simulink model "flightControlSystem"  (R2020b)
settings: Solver=ode3  StartTime=0  StopTime=TFinal  FixedStep=Ts  RelTol=1e-3  EnableMultiTasking=on
undefined symbols (not defined in the file): codertarget, Controller, DiscIntNeverNeededParam, Discrete, Estimator, g, gray, init, Rec, SDTV, Sensors, Time, Ts, var_acc_angle_N, var_bias_gyr_N, var_gyro_p_N, Vehicle
libraries: simulink x43, pid_lib x4, ctrlSharedLib x4, visiontransforms x4, sharedtransform x3, eeGeneralControl x2, visionstatistics x2, visionconversions x2, dspindex x2, dspbuff3 x1, uavalgslib x1, visiontextngfix x1
(part 3 of 3)

== system flightControlSystem/Flight Control System/State Estimator/XY Position Estimator/EstimatorXYPosition ==
  note: Switching from orientationControl to Position
      | control reset the current world position estimate
      | (happens when using no markers)
  dxy_estimin : Inport
  orient_estimin : Inport  Port=2  SampleTime=Ts
  controlModePosVSOrient_flagin : Inport  Port=3
  dz_estimin : Inport  Port=4
  Math Function : Math  Operator=transpose  SignedPower=on  SaturateOnIntegerOverflow=on
  Mux2 : Mux  Inputs=2
  Product : Product  Multiplication=Matrix(*)
  Rotation Angles to Direction Cosine Matrix : sharedtransform/Rotation Angles to Direction Cosine Matrix  rotationOrder=ZYX  aMode=aMode
      settings: SourceProductBaseCode=AE,PW,MT,UV,VE,VP
  SelectdXY : Selector  InputPortWidth=3  IndexOptions=Index vector (dialog)  Indices=[1 2]  OutputSizes=1
  SimplyIntegrateVelocity : DiscreteIntegrator  ExternalReset=rising  SampleTime=Ts  ICPrevOutput=DiscIntNeverNeededParam  ICPrevScaledInput=DiscIntNeverNeededParam
  XY_estimout : Outport  VectorParamsAs1DForOutWhenUnconnected=off
  wires:
  controlModePosVSOrient_flagin/1 -> SimplyIntegrateVelocity/2
  Product/1 -> SelectdXY/1
  Mux2/1 -> Product/2
  dz_estimin/1 -> Mux2/2
  SimplyIntegrateVelocity/1 -> XY_estimout/1
  dxy_estimin/1 -> Mux2/1
  orient_estimin/1 -> Rotation Angles to Direction Cosine Matrix/1
  Rotation Angles to Direction Cosine Matrix/1 -> Math Function/1
  SelectdXY/1 -> SimplyIntegrateVelocity/1
  Math Function/1 -> Product/1

== system flightControlSystem/Flight Control System/State Estimator/SensorPreprocessing/Temperature Compensation/Triggered Subsystem ==
  In1 : Inport
  Trigger : TriggerPort  TriggerType=either  VariantControl=Variant
  Out1 : Outport
  wires:
  In1/1 -> Out1/1

== system flightControlSystem/Flight Control System/State Estimator/XY Position Estimator/EstimatorVelocity/AccelerationHandling ==
  dxy_estimin : Inport
  sensorIMU_datin : Inport  Port=2
  orient_estimin : Inport  Port=3
  Z_estimin : Inport  Port=4
  Add : Sum  Inputs=-+
  Bus Selector1 : BusSelector  OutputSignals=ddx,ddy,ddz
  Deactivate Acceleration If OF is not used due to low altitude : simulink/Logic and Bit Operations/Compare To Constant  relop=<=  const=Estimator.pos.opticalFlowZMax  OutDataTypeStr=boolean
  Logical Operator : Logic  Operator=OR  AllPortsSameDT=off  OutDataTypeStr=boolean
  Mux6 : Mux  Inputs=3
  Product : Product  Inputs=3
  Product1 : Product  Multiplication=Matrix(*)
  Rotation Angles to Direction Cosine Matrix : sharedtransform/Rotation Angles to Direction Cosine Matrix  rotationOrder=ZYX  aMode=aMode
      settings: SourceProductBaseCode=AE,PW,MT,UV,VE,VP
  SelectPlanarddxy : Selector  InputPortWidth=3  IndexOptions=Index vector (dialog)  Indices=[1 2]  OutputSizes=1
  Selector : Selector  InputPortWidth=2  IndexOptions=Index vector (dialog)  Indices=1  OutputSizes=1
  Selector1 : Selector  InputPortWidth=2  IndexOptions=Index vector (dialog)  Indices=2  OutputSizes=1
  do not use acc if optical flow never available (Note OF@60Hz but ZOH to 200!) : simulink/Logic and Bit Operations/Compare To Constant  relop=~=  const=0  OutDataTypeStr=boolean
  do not use acc if optical flow never available (Note OF@60Hz but ZOH to 200!)1 : simulink/Logic and Bit Operations/Compare To Constant  relop=~=  const=0  OutDataTypeStr=boolean
  gainaccinput1 : Gain  OutDataTypeStr=single
  gravity : Constant  Value=[0 0 -g]
  acceleration_world : Outport  OutDataTypeStr=single  VectorParamsAs1DForOutWhenUnconnected=off
  wires:
  do not use acc if optical flow never available (Note OF@60Hz but ZOH to 200!)1/1 -> Logical Operator/2
  do not use acc if optical flow never available (Note OF@60Hz but ZOH to 200!)/1 -> Logical Operator/1
  Logical Operator/1 -> Product/1
  Selector1/1 -> do not use acc if optical flow never available (Note OF@60Hz but ZOH to 200!)1/1
  Selector/1 -> do not use acc if optical flow never available (Note OF@60Hz but ZOH to 200!)/1
  dxy_estimin/1 -> Selector1/1, Selector/1
  Product/1 -> acceleration_world/1
  Deactivate Acceleration If OF is not used due to low altitude/1 -> Product/3
  Z_estimin/1 -> Deactivate Acceleration If OF is not used due to low altitude/1
  Add/1 -> SelectPlanarddxy/1
  Product1/1 -> Add/1
  gravity/1 -> Product1/2
  SelectPlanarddxy/1 -> gainaccinput1/1
  Bus Selector1/3 -> Mux6/3  "<ddz>"
  Bus Selector1/1 -> Mux6/1  "<ddx>"
  sensorIMU_datin/1 -> Bus Selector1/1
  Mux6/1 -> Add/2
  Bus Selector1/2 -> Mux6/2  "<ddy>"
  orient_estimin/1 -> Rotation Angles to Direction Cosine Matrix/1
  Rotation Angles to Direction Cosine Matrix/1 -> Product1/1
  gainaccinput1/1 -> Product/2

== system flightControlSystem/Flight Control System/State Estimator/XY Position Estimator/EstimatorVelocity/Angular velocity compensation for optical flow ==
  note: Optical flow readings are affected by both linear and angular velocity of the drone. We need to subtract the effect of angular velocity before using the flow data
  z_estimate : Inport
  Angular velocity w/o bias : Inport  Port=2
  Abs : Abs
  Data Type Conversion : DataTypeConversion
  Demux : Demux  Outputs=2
  Gain1 : Gain  Gain=-1
  Mux : Mux  Inputs=2
  Selector : Selector  InputPortWidth=3  IndexOptions=Index vector (dialog)  Indices=[1 2]  OutputSizes=1
  prod : Product  Inputs=**
  angular velocity correction : Outport
  wires:
  Gain1/1 -> Mux/1
  Mux/1 -> Data Type Conversion/1
  Demux/2 -> Gain1/1
  Data Type Conversion/1 -> angular velocity correction/1
  prod/1 -> Demux/1
  z_estimate/1 -> Abs/1
  Demux/1 -> Mux/2
  Selector/1 -> prod/2
  Abs/1 -> prod/1
  Angular velocity w/o bias/1 -> Selector/1

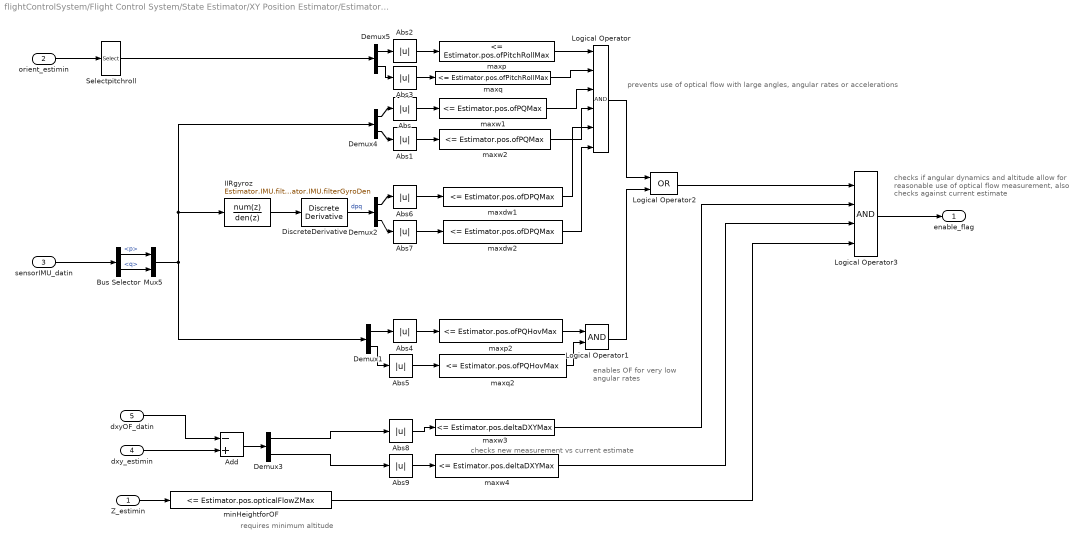
== system flightControlSystem/Flight Control System/State Estimator/XY Position Estimator/EstimatorVelocity/DataHandling ==
  note: prevents use of optical flow with large angles, angular rates or accelerations
  note: enables OF for very
      | low angular rates
  note: checks if angular dynamics and altitude allow for
      | reasonable use of optical flow measurement,
      | also checks against current estimate
  note: checks new measurement vs current estimate
  note: requires minimum altitude
  Z_estimin : Inport
  orient_estimin : Inport  Port=2
  sensorIMU_datin : Inport  Port=3
  dxy_estimin : Inport  Port=4
  dxyOF_datin : Inport  Port=5
  Abs{,1..9} (10 alike) : Abs
  Add : Sum  Inputs=-+
  Bus Selector : BusSelector  OutputSignals=p,q
  Demux{1..5} (5 alike) : Demux  Outputs=2
  DiscreteDerivative : simulink/Discrete/Discrete Derivative  gainval=1.0  ICPrevScaledInput=0.0  OutMin=[]  OutMax=[]  OutDataType=fixdt(1, 16)  OutScaling=2^-10  DoSatur=off
  IIRgyroz : DiscreteFilter  Numerator=Estimator.IMU.filterGyroNum  Denominator=Estimator.IMU.filterGyroDen
  Logical Operator : Logic  Inputs=6  AllPortsSameDT=off  OutDataTypeStr=boolean
  Logical Operator1 : Logic  AllPortsSameDT=off  OutDataTypeStr=boolean
  Logical Operator2 : Logic  Operator=OR  AllPortsSameDT=off  OutDataTypeStr=boolean
  Logical Operator3 : Logic  Inputs=4  AllPortsSameDT=off  OutDataTypeStr=boolean
  Mux5 : Mux  Inputs=2
  Selectpitchroll : Selector  InputPortWidth=3  IndexOptions=Index vector (dialog)  Indices=[2 3]  OutputSizes=1
  maxdw1 : simulink/Logic and Bit Operations/Compare To Constant  relop=<=  const=Estimator.pos.ofDPQMax  OutDataTypeStr=boolean
  maxdw2 : simulink/Logic and Bit Operations/Compare To Constant  relop=<=  const=Estimator.pos.ofDPQMax  OutDataTypeStr=boolean
  maxp : simulink/Logic and Bit Operations/Compare To Constant  relop=<=  const=Estimator.pos.ofPitchRollMax  OutDataTypeStr=boolean
  maxp2 : simulink/Logic and Bit Operations/Compare To Constant  relop=<=  const=Estimator.pos.ofPQHovMax  OutDataTypeStr=boolean
  maxq : simulink/Logic and Bit Operations/Compare To Constant  relop=<=  const=Estimator.pos.ofPitchRollMax  OutDataTypeStr=boolean
  maxq2 : simulink/Logic and Bit Operations/Compare To Constant  relop=<=  const=Estimator.pos.ofPQHovMax  OutDataTypeStr=boolean
  maxw1 : simulink/Logic and Bit Operations/Compare To Constant  relop=<=  const=Estimator.pos.ofPQMax  OutDataTypeStr=boolean
  maxw2 : simulink/Logic and Bit Operations/Compare To Constant  relop=<=  const=Estimator.pos.ofPQMax  OutDataTypeStr=boolean
  maxw3 : simulink/Logic and Bit Operations/Compare To Constant  relop=<=  const=Estimator.pos.deltaDXYMax  OutDataTypeStr=boolean
  maxw4 : simulink/Logic and Bit Operations/Compare To Constant  relop=<=  const=Estimator.pos.deltaDXYMax  OutDataTypeStr=boolean
  minHeightforOF : simulink/Logic and Bit Operations/Compare To Constant  relop=<=  const=Estimator.pos.opticalFlowZMax  OutDataTypeStr=boolean
  enable_flag : Outport  VectorParamsAs1DForOutWhenUnconnected=off
  wires:
  minHeightforOF/1 -> Logical Operator3/4
  IIRgyroz/1 -> DiscreteDerivative/1
  Mux5/1 -> Demux1/1, Demux4/1, IIRgyroz/1
  maxw4/1 -> Logical Operator3/3
  maxw3/1 -> Logical Operator3/2
  dxyOF_datin/1 -> Add/1
  Demux3/2 -> Abs9/1
  Demux3/1 -> Abs8/1
  dxy_estimin/1 -> Add/2
  Add/1 -> Demux3/1
  Abs9/1 -> maxw4/1
  Abs8/1 -> maxw3/1
  Logical Operator2/1 -> Logical Operator3/1
  Logical Operator3/1 -> enable_flag/1
  DiscreteDerivative/1 -> Demux2/1  "dpq"
  Demux2/2 -> Abs7/1
  Demux2/1 -> Abs6/1
  Abs7/1 -> maxdw2/1
  Abs6/1 -> maxdw1/1
  Logical Operator1/1 -> Logical Operator2/2
  Demux1/2 -> Abs5/1
  Demux1/1 -> Abs4/1
  Abs5/1 -> maxq2/1
  Abs4/1 -> maxp2/1
  Abs3/1 -> maxq/1
  Abs2/1 -> maxp/1
  Demux4/2 -> Abs1/1
  Demux4/1 -> Abs/1
  Abs1/1 -> maxw2/1
  Abs/1 -> maxw1/1
  Z_estimin/1 -> minHeightforOF/1
  Logical Operator/1 -> Logical Operator2/1
  maxw1/1 -> Logical Operator/3
  Bus Selector/1 -> Mux5/1  "<p>"
  Selectpitchroll/1 -> Demux5/1
  sensorIMU_datin/1 -> Bus Selector/1
  maxq2/1 -> Logical Operator1/2
  Bus Selector/2 -> Mux5/2  "<q>"
  maxp/1 -> Logical Operator/1
  maxw2/1 -> Logical Operator/4
  orient_estimin/1 -> Selectpitchroll/1
  maxdw1/1 -> Logical Operator/5
  maxdw2/1 -> Logical Operator/6
  maxq/1 -> Logical Operator/2
  Demux5/1 -> Abs2/1
  Demux5/2 -> Abs3/1
  maxp2/1 -> Logical Operator1/1

== system flightControlSystem/Flight Control System/State Estimator/XY Position Estimator/EstimatorVelocity/XY velocity w//o angular velocity compensation ==
  note: Optical flow raw readings are converted to velocity in m/s based on the estimated altitude
  optical_flow : Inport
  z_estimate : Inport  Port=2
  " " : Product  Inputs=**
  Compare To Constant : simulink/Logic and Bit Operations/Compare To Constant  relop=<  const=200*4  OutDataTypeStr=boolean
  Counter Free-Running : simulink/Sources/Counter Free-Running  NumBits=32  tsamp=-1
  Gain : Gain  Gain=-1
  Select dxy : Selector  InputPortWidth=3  IndexOptions=Index vector (dialog)  Indices=[1 2]  OutputSizes=1
  Switch : Switch  Criteria=u2 > Threshold
  opticalFlowErrorCorrect : Gain  Gain=1.15
  optical_flow_dx_dy : Outport
  wires:
  Select dxy/1 -> optical_flow_dx_dy/1  "optical_flow_dx_dy"
  " "/1 -> opticalFlowErrorCorrect/1
  opticalFlowErrorCorrect/1 -> Switch/3
  Gain/1 -> " "/2
  Switch/1 -> Select dxy/1
  Counter Free-Running/1 -> Compare To Constant/1
  Compare To Constant/1 -> Switch/2
  optical_flow/1 -> " "/1, Switch/1
  z_estimate/1 -> Gain/1

== matlab function flightControlSystem/Image Processing System/MATLAB Function ==
  data: lines_struc input; x output; y output
function [x,y]  = create_line_matrix(lines_struc)
    % convert lines struct to matrix
    coder.varsize('lines');
    lines = zeros(20,6);
    if size(lines_struc,1)<=20
        for i=1:size(lines_struc,1)
            lines(i,1) = lines_struc(i,1);
            lines(i,2) = lines_struc(i,2);
            lines(i,3) = lines_struc(i,3);
            lines(i,4) = lines_struc(i,4);
            line_vector = [lines(i,3)-lines(i,1), lines(i,4)-lines(i,2)];
            angle_slop = calculate_slop_angle(line_vector);
            lines(i,5) = angle_slop;
            lines(i,6) = sqrt((lines(i,3)-lines(i,1))^2+(lines(i,4)-lines(i,2))^2);
        end
    else
        for i=1:20
            lines(i,1) = lines_struc(i,1);
            lines(i,2) = lines_struc(i,2);
            lines(i,3) = lines_struc(i,3);
            lines(i,4) = lines_struc(i,4);
            line_vector = [lines(i,3)-lines(i,1), lines(i,4)-lines(i,2)];
            angle_slop = calculate_slop_angle(line_vector);
            lines(i,5) = angle_slop;
            lines(i,6) = sqrt((lines(i,3)-lines(i,1))^2+(lines(i,4)-lines(i,2))^2);
        end
    end
    
    %delete short line
    short_line_index = find(lines(:,6)<15);
    all_index = [1:1:20];
    all_index = all_index';
    long_line_index = setdiff(all_index,short_line_index,'rows');
    nline = size(long_line_index,1);
    new_lines = zeros(nline,6);
    new_lines = lines(long_line_index,:);
    lines = new_lines;
    %
    
    % detect lines to merge
    coder.varsize('parallel_line');
    parallel_line = zeros(20,8);
    parallel_line_insert_idx = 1;
    slop_value = unique(lines(:,5)); %OK
    coder.varsize('slop_value_to_checkmerge');
    slop_value_to_checkmerge = zeros(20,1); 
    slop_value_to_checkmerge_insert_idx = 1;
    coder.varsize('checked_slop');
    checked_slop = zeros(20,1);
    checked_slop_insert_idx = 1;
    if size(slop_value,1)>0
        for j = 1:size(slop_value,1)
            slop = slop_value(j);
            index_lines = find(abs(lines(:,5)-slop)<10);
            if size(index_lines,1)==2 && ~any(ismember(lines(index_lines,5),checked_slop))
                parallel_line(parallel_line_insert_idx,1:8) = [lines(index_lines(1),1:4),lines(index_lines(2),1:4)];
                parallel_line_insert_idx = parallel_line_insert_idx + 1 ;
            elseif size(index_lines,1)>2 && ~any(ismember(lines(index_lines,5),checked_slop))
                slop_value_to_checkmerge(slop_value_to_checkmerge_insert_idx) = slop;
                slop_value_to_checkmerge_insert_idx = slop_value_to_checkmerge_insert_idx+1;
            end
            checked_slop(checked_slop_insert_idx) = slop;
            checked_slop_insert_idx = checked_slop_insert_idx+1;
        end
    end
    slop_value_to_checkmerge = find(slop_value_to_checkmerge(:)~=0);
    %

    possible_interdistance = 100;
    if size(slop_value_to_checkmerge,1)>0
        for j=1:size(slop_value_to_checkmerge,1)
            slop = slop_value_to_checkmerge(j);
            index_lines = find(abs(lines(:,5)-slop)<10);
            %index_lines (maybe not only 2)
            middle_point_coordinates = [(lines(index_lines,1)+lines(index_lines,3))/2, (lines(index_lines,2)+lines(index_lines,4))/2];
            coder.varsize('merge_line_idx');
            merge_line_idx = zeros(20,2);
            merge_line_insert_idx = 1;
            for k=1:size(middle_point_coordinates,1)-1
                for h=k+1:size(middle_point_coordinates,1)
                    p1 = middle_point_coordinates(k,:);
                    p2 = middle_point_coordinates(h,:);
                    middle_slop_vector = [(p1(2)-p2(2)),p1(1)-p2(1)];
                    middle_slop = calculate_slop_angle(middle_slop_vector);
                    if abs(middle_slop-slop)<10
                        %note down line index to merge
                        merge_line_idx(merge_line_insert_idx,:) = [index_lines(k),index_lines(h)];
                        merge_line_insert_idx = merge_line_insert_idx+1;
                    end
                end
            end
            merge_line_idx = merge_line_idx(find(any(merge_line_idx,2)),:);
            remained_line_idx = index_lines(~ismember(index_lines(:),merge_line_idx(:)));
            coder.varsize('after_merged_lines');
            after_merged_lines = zeros(20,6);
            after_merged_lines(1:size(remained_line_idx,1),1:4) = lines(remained_line_idx,1:4);
            after_merged_lines_insert_idx = size(remained_line_idx,1)+1;
            
            
            while(size(merge_line_idx,1)>0)
                coder.varsize('merge_idx_tmp');
                merge_idx_tmp = zeros(20,1);
                merge_idx_tmp(1) = merge_line_idx(1,1); 
                merge_idx_tmp(2) = merge_line_idx(1,2);
                merge_idx_tmp_insert_idx = 3;
                line_to_delete_in_merge_line_idx = zeros(size(merge_line_idx,1),1);
                line_to_delete_in_merge_line_idx(1) = 1;
                line_to_delete_in_merge_line_idx_insert_idx = 2;
                if (size(merge_line_idx,1)>1)
                    for i=2:size(merge_line_idx,1)
                        if ismember(merge_line_idx(i,1),merge_idx_tmp)
                            merge_idx_tmp(merge_idx_tmp_insert_idx) = merge_line_idx(i,2);
                            merge_idx_tmp_insert_idx = merge_idx_tmp_insert_idx+1;
                            line_to_delete_in_merge_line_idx(line_to_delete_in_merge_line_idx_insert_idx) = i;
                            line_to_delete_in_merge_line_idx_insert_idx = line_to_delete_in_merge_line_idx_insert_idx+1;
                        elseif ismember(merge_line_idx(i,2),merge_idx_tmp)
                            merge_idx_tmp(merge_idx_tmp_insert_idx) = merge_line_idx(i,1);
                            merge_idx_tmp_insert_idx = merge_idx_tmp_insert_idx+1;
                            line_to_delete_in_merge_line_idx(line_to_delete_in_merge_line_idx_insert_idx) = i;
                            line_to_delete_in_merge_line_idx_insert_idx = line_to_delete_in_merge_line_idx_insert_idx+1;
                        end
                    end
                end
                merge_idx_tmp = merge_idx_tmp(find(any(merge_idx_tmp,2)),:);
                line_to_delete_in_merge_line_idx = line_to_delete_in_merge_line_idx(find(any(line_to_delete_in_merge_line_idx,2)),:);
                % operations on lines_copy
                coordinates_to_merge = lines(merge_idx_tmp',1:4);
                coordinates_to_merge = [coordinates_to_merge(:,1:2);coordinates_to_merge(:,3:4)];
                % find farest point among all coordinates
                npoint = size(coordinates_to_merge,1);
                longest_length =0;
                node = zeros(1,4);
                for k=1:npoint-1
                    for h=k+1:npoint
                       test_length = sqrt((coordinates_to_merge(k,1)-coordinates_to_merge(h,1))^2+(coordinates_to_merge(k,2)-coordinates_to_merge(h,2))^2);
                       if test_length>longest_length
                           longest_length = test_length;
                           node(1,1:4) = [coordinates_to_merge(k,:),coordinates_to_merge(h,:)];
                       end
                    end
                end
                after_merged_lines(after_merged_lines_insert_idx,1:4) = node;
                after_merged_lines_insert_idx = after_merged_lines_insert_idx+1;
                % operations on merge_line_idx
                merge_line_idx_remain_lines = setdiff([1:1:size(merge_line_idx,1)],line_to_delete_in_merge_line_idx);
                merge_line_idx = merge_line_idx(merge_line_idx_remain_lines,:); 
            end
            % from after_merged_lines, form pairs of parallel lines
            % set after_merge_lines column x1 y1 x2 y2 m_x m_y
            after_merged_lines(:,5) = (after_merged_lines(:,1)+after_merged_lines(:,3))/2;
            after_merged_lines(:,6) = (after_merged_lines(:,2)+after_merged_lines(:,4))/2;
            while (size(after_merged_lines,1)/2>1) %match paralle lines
               p1_tt = after_merged_lines(1,1:2);
               p2_tt = after_merged_lines(1,3:4);
               p3_tt = after_merged_lines(1,5:6);
               other_points = [after_merged_lines(2:end,1:2); after_merged_lines(2:end,3:4); after_merged_lines(2:end,5:6)];
               n_other_lines = size(other_points,1)/3;
               angles = zeros(size(other_points,1),1); %%%
               angles_insert_idx = 1;
               for i=1:size(other_points,1)
                   s1v = [other_points(i,1)-p1_tt(1),other_points(i,2)-p1_tt(2)];
                   s2v = [other_points(i,1)-p2_tt(1),other_points(i,2)-p2_tt(2)];
                   s3v = [other_points(i,1)-p3_tt(1),other_points(i,2)-p3_tt(2)];
                   s1 = calculate_slop_angle(s1v);
                   s2 = calculate_slop_angle(s2v);
                   s3 = calculate_slop_angle(s3v);
                   diff1 = abs(abs(s1-slop)-90);
                   diff2 = abs(abs(s2-slop)-90);
                   diff3 = abs(abs(s3-slop)-90);
                   D = [diff1, diff2, diff3];
                   angles(angles_insert_idx) = min(D);
                   angles_insert_idx = angles_insert_idx +1;
                   if min(D)<5
                       ds = [norm(s1v), norm(s2v), norm(s3v)];
                       if min(ds) < possible_interdistance && min(ds)~=0
                           possible_interdistance = min(ds);
                       end
                   end
               end
               match_idx = ceil(find(angles(:)==min(angles),1)/3)+1;
               parallel_line(parallel_line_insert_idx,1:8) = [after_merged_lines(1,1:4),after_merged_lines(match_idx,1:4)];
               parallel_line_insert_idx = parallel_line_insert_idx+1;
               after_merged_lines(1,:) = [0,0,0,0,0,0];
               after_merged_lines(match_idx,:) = [0,0,0,0,0,0];
               after_merged_lines = after_merged_lines(find(any(after_merged_lines,2)),:);
               
            end
            if size(after_merged_lines,1)==2
                parallel_line(parallel_line_insert_idx,1:8) = [after_merged_lines(1,1:4),after_merged_lines(2,1:4)];
            end
        end
    end

   
    waypoint_mx = (parallel_line(:,1)+parallel_line(:,3)+parallel_line(:,5)+parallel_line(:,7))/4;
    waypoint_my = (parallel_line(:,2)+parallel_line(:,4)+parallel_line(:,6)+parallel_line(:,8))/4;
    waypoints = zeros(size(waypoint_mx,1),3);
    waypoints(:,1:2) = [waypoint_mx, waypoint_my;];
    scaling = 0.05/possible_interdistance;
    waypoints_valid = waypoints.*scaling;
    %exclude behind point
    origin = [120, 80];
    for i=1:size(waypoints,1)
        if waypoints(i,2)>origin(2)
            waypoints_valid(i,:) = [0,0,0];
        end
    end
    idx_valid_waypoints = find(any(waypoints_valid,2));
    waypoints_valid = waypoints_valid(idx_valid_waypoints,:);
    waypoints = waypoints(idx_valid_waypoints,:);

    %exclude close point
    for i=1:size(waypoints,1)-1
        for j=i+1:size(waypoints,1)
            d = sqrt((waypoints_valid(i,1)-waypoints_valid(j,1))^2+(waypoints_valid(i,2)-waypoints_valid(j,2))^2);
            if d<0.05
                waypoints_valid(j,:) = [0,0,0];
            end
        end
    end

    idx_valid_waypoints = find(any(waypoints_valid,2));
    waypoints_valid = waypoints_valid(idx_valid_waypoints,:);
    waypoints = waypoints(idx_valid_waypoints,:);

    %order waypoints

    for i=1:size(waypoints,1)
        d_to_origin = sqrt((waypoints(i,1)-origin(1))^2+(waypoints(i,2)-origin(2))^2);
        waypoints(i,3) = d_to_origin;
    end
    [out,idx] = sort(waypoints(:,3));
    waypoints_valid = waypoints_valid(idx,:);
    if size(waypoints_valid,1)>0 && size(waypoints_valid,2)>0
        x = waypoints_valid(1,1);
        y = waypoints_valid(1,2);
    else
        x = 0;
        y = 0;
    end
end

function [slop_angle] = calculate_slop_angle(v)
    horizontal_vector = [50,0];
    x1 = horizontal_vector(1);
    y1 = horizontal_vector(2);
    x2 = v(1);
    y2 = v(2);
    slop_angle = atan2d(x1*y2-y1*x2,x1*x2+y1*y2);
end

== matlab function flightControlSystem/Flight Control System/Controller/Position Controller/Position error transformation (Earth to Body frame) ==
  data: yaw input; xy_err_earth input; xy_err_body output
function xy_err_body = fcn(yaw,xy_err_earth)

transformation = [cos(yaw), sin(yaw); -sin(yaw),  cos(yaw)];
xy_err_body = transformation * xy_err_earth;


end

== matlab function flightControlSystem/Flight Control System/Path Planning/Subsystem1/MATLAB Function ==
  data: x input; stop_command output; y input; next_delta output size=[1 3]; hover_longtime input; hover_flag output
function [stop_command, next_delta, hover_flag] = fcn(x,y,hover_longtime)
    next_delta = zeros(1,3);
    if size(x,1)<1 && size(y,1)<1
        next_delta(1,1) = 0;
        next_delta(1,2) = 0;
        next_delta(1,3) = 0;
        hover_flag = 1;
    else
        next_delta(1,1) = x;
        next_delta(1,2) = y;
        hover_flag = 0;
    end
    if hover_longtime
        stop_command = 1;
    else
        stop_command = 0;
    end
    
    
end
% waypoint should never be 0 0 0 otherwise error of non continuity 
%     if (size(x,1)==0 && size(y,1)==0)
%         stop_command = 0;
%         next_waypoint(1,1) = accumulated_x+0;
%         next_waypoint(1,2) = accumulated_y+0;
%         next_waypoint(1,3) = -0.7;
%         cas = 1;
%     elseif (size(x,1)>0 && size(y,1)>0 && x(end)==0 && y(end)==0 )
%         stop_command = 0;%1
%         next_waypoint(1,1) = accumulated_x;
%         next_waypoint(1,2) = accumulated_y;
%         next_waypoint(1,3) = -0.7;
%         cas = 2;
%     else
%         x_old = accumulated_x;
%         y_old = accumulated_y;
%         next_waypoint(1,1) = x_old + x(end);
%         next_waypoint(1,2) = y_old + y(end);
%         next_waypoint(1,3) = -0.7;
%         stop_command = 0;
%         cas = 3;
%     end

== matlab function flightControlSystem/Image Processing System/MATLAB Function1 ==
  data: BW input; BW output
function BW = fcn(BW)
    BW = imclose(BW, strel('disk',2));
    BW = bwmorph(BW, 'skel', 40);
end

== matlab function flightControlSystem/Image Processing System/MATLAB Function2 ==
  data: pts input; x output; y output
function [x,y] = fcn(pts)
    %drone_position = [120 80];
    scaling_horizontal = 0.0037; % m/pixel
    scaling_vertical = 0.0035;
    x1 = double(pts(1,1));
    y1 = double(pts(1,2));
    x2 = double(pts(2,1));
    y2 = double(pts(2,2));
    x3 = double(pts(3,1));
    y3 = double(pts(3,2));
    x4 = double(pts(4,1));
    y4 = double(pts(4,2));
    
    % verify zero lines
    zeros_flag = any(pts,2);
    n_zero_line = nnz(zeros_flag);
    waypoints_raw = zeros(2,2);
    waypoints = zeros(2,2);
    if n_zero_line==0
        %end waypoint computation, no line detected
        waypoints_raw = [107,107; 107,107];
    elseif n_zero_line==2
        idx = find(zeros_flag(:)~=0);
        if isequal(idx, [1;2])
            waypoints_raw = [x1, y1; (x1+x2)/2, (y1+y2)/2;];
        else
            waypoints_raw = [x3, y3; (x3+x4)/2, (y3+y4)/2;];
        end
    else
        tail_plat = find(pts(:,2)==0);
        if size(tail_plat,1)==2
            waypoints_raw = [sum(pts(tail_plat,1))/2,sum(pts(tail_plat,2))/2; sum(pts(tail_plat,1))/2,sum(pts(tail_plat,2))/2; ];
            scaling_horizontal = 0;
        else
            waypoints_raw = [(x1+x3)/2, (y1+y3)/2; (x1+x2+x3+x4)/4, (y1+y2+y3+y4)/4];
        end
    end
    waypoints_raw(:,1) = waypoints_raw(:,1)-107;
    waypoints_raw(:,2) = waypoints_raw(:,2)-107;
    if size(find(waypoints_raw(:,2)>0),1)
        n_setzeros = size(find(waypoints_raw(:,2)>0),1);
        waypoints_raw(find(waypoints_raw(:,2)>0),1:2) = zeros(n_setzeros,2);
    end
    waypoints(:,1) = waypoints_raw(:,1)*scaling_horizontal;
    waypoints(:,2) = waypoints_raw(:,2)*scaling_vertical;
    distance1 = sqrt(waypoints(1,1)^2+waypoints(1,2)^2);
    distance2 = sqrt(waypoints(2,1)^2+waypoints(2,2)^2);
    if distance1>distance2
        y = waypoints(2,1);
        x = -1 * waypoints(2,2);
        
    else
        y = waypoints(1,1);
        x = -1 * waypoints(1,2);
        
    end
% x y parameter need change frame
    
end

== matlab function flightControlSystem/Flight Control System/Path Planning/Waypoint follower/MATLAB Function ==
  data: position input; next_x output; delta_pos input; flag input; old_target input; next_y output; next_z output
function [next_x, next_y, next_z]  = fcn(position,delta_pos,flag,old_target)
    next_x = 0;
    next_y = 0;
    next_z = 0;
    if flag ==1
        
        next_x = position(1,1)+delta_pos(1,1);
        next_y = position(2,1)+delta_pos(1,2);
        next_z = position(3,1)+delta_pos(1,3);
    else
        next_x = old_target(1,1);
        next_y = old_target(2,1);
        next_z = old_target(3,1);
    end
end

== matlab function flightControlSystem/Flight Control System/Path Planning/Waypoint follower/MATLAB Function1 ==
  data: next_x input; next_y input; next_z input; complete_flag output; position input
function complete_flag   = fcn(next_x, next_y, next_z,position)
    if abs(next_x-position(1,1))>0.02 && abs(next_y-position(2,1))>0.02
        complete_flag = 0;
        
    else
        complete_flag = 1;
    end
end
